simulink model "Evaporator"  (R2022b)
settings: Solver=VariableStepAuto  StartTime=0.0  StopTime=10.0  RelTol=1e-3
settings Model: Creator=YJT  LastModifiedBy=YJT
settings SolverCC: AlgebraicLoopSolver=TrustRegion
settings DebuggingCC: UnconnectedInputMsg=warning  UnconnectedOutputMsg=warning  UnconnectedLineMsg=warning  SFMachineParentedDataDiag=warning
settings ModelReferenceCC: EnableRefExpFcnMdlSchedulingChecks=on

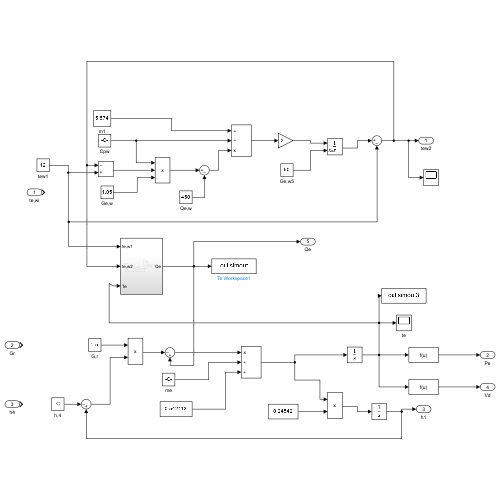
[thumbnail: Simulink's stored preview of the top-level diagram]
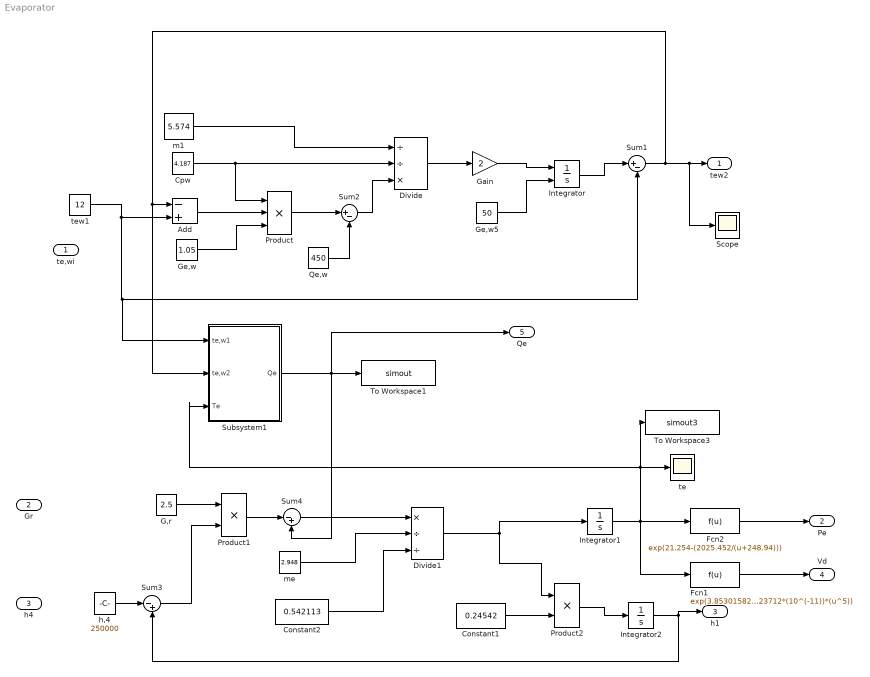
== system Evaporator ==
  te,wi : Inport
  Gr : Inport  Port=2
  h4 : Inport  Port=3
  Add : Sum  Inputs=-+
  Constant1 : Constant  Value=0.24542
  Constant2 : Constant  Value=0.542113
  Cpw : Constant  Value=4.187
  Divide : Product  Inputs=//*
  Divide1 : Product  Inputs=*//
  Fcn1 : Fcn  Expr=exp(3.85301582-3.1563*(10^(-2))*u+10.3312754*(10^(-5))*(u^2)-6.27787965*(10^(-7))*(u^3)+1.37486693*(10^(-9))*(u^4)-2.07723712*(10^(-11))*(u^5))
  Fcn2 : Fcn  Expr=exp(21.254-(2025.452/(u+248.94)))
  G,r : Constant  Value=2.5
  Gain : Gain  Gain=2
  Ge,w : Constant  Value=1.05
  Ge,w5 : Constant  Value=50
  Integrator : Integrator  InitialConditionSource=external
  Integrator1 : Integrator
  Integrator2 : Integrator
  Product : Product  Inputs=3
  Product1 : Product
  Product2 : Product
  Qe,w : Constant  Value=450
  Scope : Scope
  Subsystem1 : Subsystem
  Sum1 : Sum  Inputs=|+-
  Sum2 : Sum  Inputs=|+-
  Sum3 : Sum  Inputs=|-+
  Sum4 : Sum  Inputs=|-+
  To Workspace1 : ToWorkspace  VariableName=simout  SaveFormat=Timeseries  SampleTime=-1
  To Workspace3 : ToWorkspace  VariableName=simout3  SaveFormat=Timeseries  SampleTime=-1
  h,4 : Constant  Value=250000
  m1 : Constant  Value=5.574
  me : Constant  Value=2.948
  te : Scope
  tew1 : Constant  Value=12
  tew2 : Outport
  Pe : Outport  Port=2
  h1 : Outport  Port=3
  Vd : Outport  Port=4
  Qe : Outport  Port=5
  wires:
  Add/1 -> Product/2
  Ge,w/1 -> Product/3
  Cpw/1 -> Product/1, Divide/2
  m1/1 -> Divide/1
  Product/1 -> Sum2/1
  Sum2/1 -> Divide/3
  Divide/1 -> Gain/1
  Gain/1 -> Integrator/1
  Integrator/1 -> Sum1/1
  Sum1/1 -> Subsystem1/2(te,w2), Add/1, Scope/1, tew2/1
  Sum3/1 -> Product1/2
  Product1/1 -> Sum4/1
  Sum4/1 -> Divide1/1
  me/1 -> Divide1/2
  Constant2/1 -> Divide1/3
  Constant1/1 -> Product2/2
  Divide1/1 -> Integrator1/1, Product2/1
  Product2/1 -> Integrator2/1
  Integrator2/1 -> h1/1, Sum3/2
  Fcn2/1 -> Pe/1
  Integrator1/1 -> Fcn1/1, te/1, Subsystem1/3(Te), To Workspace3/1, Fcn2/1
  Fcn1/1 -> Vd/1
  Subsystem1/1(Qe) -> Sum4/2, Qe/1, To Workspace1/1
  tew1/1 -> Subsystem1/1(te,w1), Sum1/2, Add/2
  Qe,w/1 -> Sum2/2
  G,r/1 -> Product1/1
  h,4/1 -> Sum3/1
  Ge,w5/1 -> Integrator/2

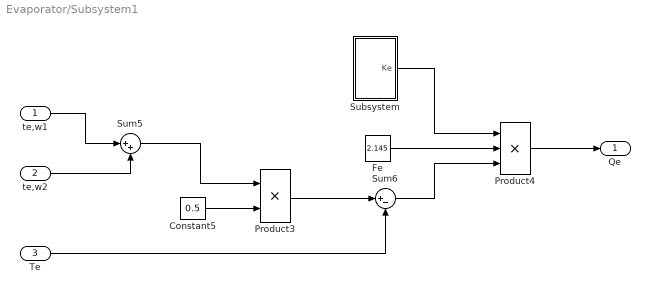
== system Evaporator/Subsystem1 ==
  te,w1 : Inport
  te,w2 : Inport  Port=2
  Te : Inport  Port=3
  Constant5 : Constant  Value=0.5
  Fe : Constant  Value=2.145
  Product3 : Product
  Product4 : Product  Inputs=3
  Subsystem : Subsystem
  Sum5 : Sum  Inputs=|++
  Sum6 : Sum  Inputs=|+-
  Qe : Outport
  wires:
  Product4/1 -> Qe/1
  Subsystem/1(Ke) -> Product4/1
  te,w2/1 -> Sum5/2
  Product3/1 -> Sum6/1
  Fe/1 -> Product4/2
  Sum6/1 -> Product4/3
  Te/1 -> Sum6/2
  Constant5/1 -> Product3/2
  Sum5/1 -> Product3/1
  te,w1/1 -> Sum5/1

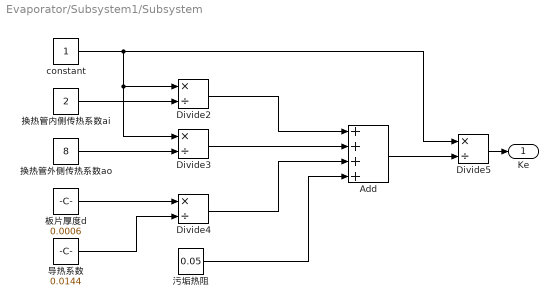
== system Evaporator/Subsystem1/Subsystem ==
  Add : Sum  Inputs=++++
  Divide{2..5} (4 alike) : Product  Inputs=*/
  constant : Constant
  导热系数 : Constant  Value=0.0144
  换热管内侧传热系数ai : Constant  Value=2
  换热管外侧传热系数ao : Constant  Value=8
  板片厚度d : Constant  Value=0.0006
  污垢热阻 : Constant  Value=0.05
  Ke : Outport
  wires:
  constant/1 -> Divide5/1, Divide2/1, Divide3/1
  导热系数/1 -> Divide4/2
  Divide3/1 -> Add/2
  污垢热阻/1 -> Add/4
  换热管内侧传热系数ai/1 -> Divide2/2
  板片厚度d/1 -> Divide4/1
  Divide2/1 -> Add/1
  换热管外侧传热系数ao/1 -> Divide3/2
  Add/1 -> Divide5/2
  Divide4/1 -> Add/3
  Divide5/1 -> Ke/1
